simulink model "radioservice"  (R2015b)
settings: Solver=FixedStepDiscrete  StartTime=0.0  StopTime=10  RelTol=1e-3
libraries: dspsigops x4, dspvision x1, dspmisc x1, dspsnks4 x1
settings Model: Creator=Shravankumar147  LastModifiedBy=Shravankumar147
settings DebuggingCC: MultiTaskRateTransMsg=warning

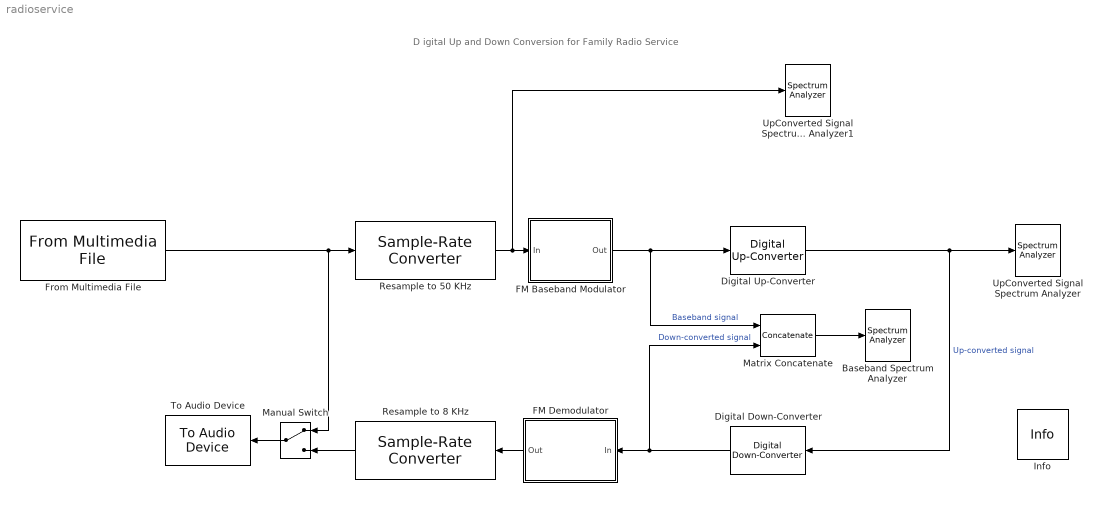
== system radioservice ==
  note: D igital Up and Down Conversion for Family Radio Service
  Baseband Spectrum Analyzer : SpectrumAnalyzer
  Digital Down-Converter : dspsigops/Digital Down-Converter  DecimationFactor=40  MinimumOrderDesign=on  NumCICSections=3  SecondFilterOrder=12  ThirdFilterOrder=10  Bandwidth=12.5e3  StopbandFrequencySource=Property  StopbandFrequency=18.75e3  PassbandRipple=0.05  StopbandAttenuation=60  Oscillator=Sine wave  CenterFrequency=455e3  NumAccumulatorBits=16  NumQuantizedAccumulatorBits=12  Dither=on  NumDitherBits=4  InheritSampleRate=on  SampleRate=30000000  outputMin=[]  outputMax=[]  SimulateUsing=Code generation
  Digital Up-Converter : dspsigops/Digital Up-Converter  InterpolationFactor=40  MinimumOrderDesign=on  FirstFilterOrder=10  SecondFilterOrder=12  NumCICSections=3  Bandwidth=12.5e3  StopbandFrequencySource=Property  StopbandFrequency=18.75e3  PassbandRipple=0.05  StopbandAttenuation=60  Oscillator=Sine wave  CenterFrequency=455e3  NumAccumulatorBits=16  NumQuantizedAccumulatorBits=12  Dither=on  NumDitherBits=4  InheritSampleRate=on  SampleRate=300000  outputMin=[]  outputMax=[]  SimulateUsing=Code generation
  FM Baseband Modulator : Subsystem
  FM Demodulator : Subsystem
  From Multimedia File : dspvision/From Multimedia File  inputFilename=speech_dft_8kHz.wav  loop=on  numPlays=inf  outputStreams=Audio only  videoDataType=single  audioDataType=double  inheritSampleTime=on  userDefinedSampleTime=1/30  noAudioOutput=off  isIntensityVideo=off  fourcc=RGB  colorVideoFormat=Separate color signals  outputEOF=off  dataOrg=Column-major  audioFrameSize=1000  computeAudioFrameSize=off  outSamplingMode=Sample based
  Info : dspmisc/Info  SystemSampleTime=-1
  Manual Switch : ManualSwitch
  Matrix Concatenate : Concatenate  Mode=Multidimensional array  ConcatenateDimension=2
  Resample to 50 KHz : dspsigops/Sample-Rate Converter  InputSampleRate=8e3  OutputSampleRate=50e3  OutputRateTolerance=0  Bandwidth=6.25e3  StopbandAttenuation=80  SimulateUsing=Code generation
  Resample to 8 KHz : dspsigops/Sample-Rate Converter  InputSampleRate=50e3  OutputSampleRate=8e3  OutputRateTolerance=0  Bandwidth=6.25e3  StopbandAttenuation=80  SimulateUsing=Code generation
  To Audio Device : dspsnks4/To Audio Device  deviceName=Default  inheritSampleRate=on  sampleRate=44100  deviceDatatype=Determine from input data type  autoBufferSize=on  bufferSize=4096  queueDuration=1.0  defaultOutputChannelMapping=on  outputChannelMapping=1:2  outputNumUnderrunSamples=off
  UpConverted Signal Spectrum Analyzer : SpectrumAnalyzer
  UpConverted Signal Spectrum Analyzer1 : SpectrumAnalyzer
  wires:
  Digital Up-Converter/1 -> Digital Down-Converter/1, UpConverted Signal Spectrum Analyzer/1  "Up-converted signal"
  Digital Down-Converter/1 -> Matrix Concatenate/2, FM Demodulator/1(In)  "Down-converted signal"
  Matrix Concatenate/1 -> Baseband Spectrum Analyzer/1
  From Multimedia File/1 -> Resample to 50 KHz/1, Manual Switch/1
  Resample to 50 KHz/1 -> UpConverted Signal Spectrum Analyzer1/1, FM Baseband Modulator/1(In)
  FM Baseband Modulator/1(Out) -> Digital Up-Converter/1, Matrix Concatenate/1  "Baseband signal"
  FM Demodulator/1(Out) -> Resample to 8 KHz/1
  Manual Switch/1 -> To Audio Device/1
  Resample to 8 KHz/1 -> Manual Switch/2

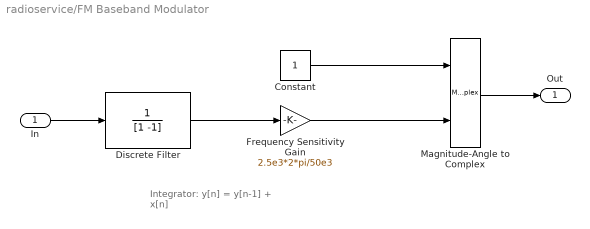
== system radioservice/FM Baseband Modulator ==
  note: Integrator:
      | y[n] = y[n-1] + x[n]
  In : Inport
  Constant : Constant  SampleTime=6250/50e3
  Discrete Filter : DiscreteFilter  Numerator=1  Denominator=[1 -1]  InputProcessing=Columns as channels (frame based)  FilterStructure=Direct form II transposed  a0EqualsOne=on
  Frequency Sensitivity Gain : Gain  Gain=2.5e3*2*pi/50e3
  Magnitude-Angle to Complex : MagnitudeAngleToComplex
  Out : Outport
  wires:
  Frequency Sensitivity Gain/1 -> Magnitude-Angle to Complex/2
  Discrete Filter/1 -> Frequency Sensitivity Gain/1
  In/1 -> Discrete Filter/1
  Magnitude-Angle to Complex/1 -> Out/1
  Constant/1 -> Magnitude-Angle to Complex/1

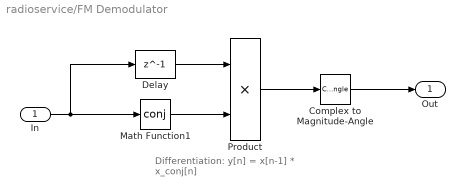
== system radioservice/FM Demodulator ==
  note: Differentiation:
      | y[n] = x[n-1] * x_conj[n]
  In : Inport
  Complex to Magnitude-Angle : ComplexToMagnitudeAngle  Output=Angle
  Delay : Delay  DelayLength=1  InitialCondition=0  InputProcessing=Columns as channels (frame based)
  Math Function1 : Math  Operator=conj  SaturateOnIntegerOverflow=on
  Product : Product  RndMeth=Zero
  Out : Outport
  wires:
  Complex to Magnitude-Angle/1 -> Out/1
  Math Function1/1 -> Product/2
  In/1 -> Math Function1/1, Delay/1
  Delay/1 -> Product/1
  Product/1 -> Complex to Magnitude-Angle/1
